simulink model "StudentClient_R2019b"  (R2019b)
settings: Solver=ode45  SolverName=VariableStepAuto  StartTime=0.0  StopTime=inf  FixedStep=1  RelTol=1e-3
undefined symbols (not defined in the file): f, gray
libraries: instrumentlib x3
settings Model: Creator=花舞  LastModifiedBy=admin
settings OptimizationCC: OptimizeBlockIOStorage=off  OptimizeDataStoreBuffers=off  BusAssignmentInplaceUpdate=off
settings DebuggingCC: SFUnexpectedBacktrackingDiag=warning  SFNoUnconditionalDefaultTransitionDiag=warning
settings RTWCC: GenerateReport=on  BuildConfiguration=Debug  LaunchReport=on
settings CodeAppCC: ForceParamTrailComments=on  MATLABSourceComments=on  EnableCustomComments=on
settings GRTTargetCC: CombineSignalStateStructs=on  SupportVariableSizeSignals=on  MultiInstanceErrorCode=Warning

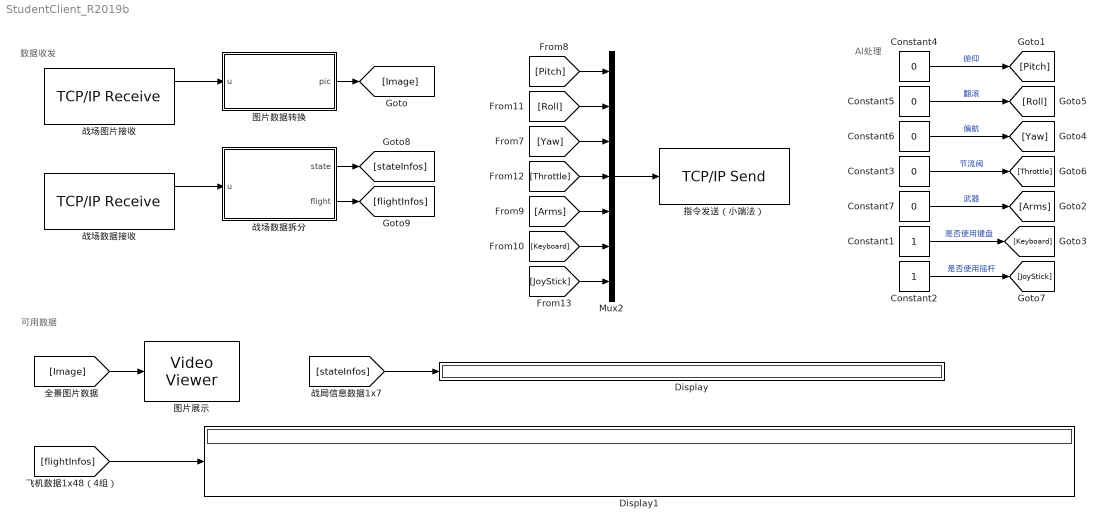
== system StudentClient_R2019b ==
  note: AI处理
  note: 可用数据
  note: 数据收发
  Constant1 : Constant  OutDataTypeStr=int32
  Constant2 : Constant  OutDataTypeStr=int32
  Constant{3..7} (5 alike) : Constant  Value=0  OutDataTypeStr=int32
  Display : Display
  Display1 : Display
  Mux2 : Mux  Inputs=7
  图片展示 : VideoViewer  colormapValue=gray(256)  FigPos=[1 1038 1920 937]
  图片数据转换 : MATLAB Function  TreatAsAtomicUnit=on
  战场图片接收 : instrumentlib/TCP//IP Receive  Host=0.0.0.0  Port=9999  DataSize="[1  1572864]"  EnableBlockingMode=off  Timeout=10  SampleTime=0.01  DataType=uint8  ByteOrder=BigEndian  ASCIIFormatting=%f,  Terminator=LF
  战场数据拆分 : MATLAB Function  TreatAsAtomicUnit=on
  战场数据接收 : instrumentlib/TCP//IP Receive  Host=0.0.0.0  Port=10000  DataSize="[1  55]"  EnableBlockingMode=off  Timeout=10  SampleTime=0.01  DataType=int32  ByteOrder=LittleEndian  ASCIIFormatting=%f,  Terminator=LF
  指令发送（小端法） : instrumentlib/TCP//IP Send  Host=0.0.0.0  Port=9999  EnableBlockingMode=off  Timeout=10  ByteOrder=LittleEndian  TransferDelay=on
  wires:
  战场图片接收/1 -> 图片数据转换/1(u)
  Constant4/1 -> [Pitch]  "俯仰"
  Constant5/1 -> [Roll]  "翻滚"
  Constant6/1 -> [Yaw]  "偏航"
  Constant3/1 -> [Throttle]  "节流阀"
  Constant7/1 -> [Arms]  "武器"
  Constant1/1 -> [Keyboard]  "是否使用键盘"
  Constant2/1 -> [JoyStick]  "是否使用摇杆"
  [Keyboard] -> Mux2/6
  [Roll] -> Mux2/2
  [Pitch] -> Mux2/1
  [Throttle] -> Mux2/4
  [Yaw] -> Mux2/3
  [Arms] -> Mux2/5
  [JoyStick] -> Mux2/7
  Mux2/1 -> 指令发送（小端法）/1
  图片数据转换/1(pic) -> [Image]
  [Image] -> 图片展示/1
  [stateInfos] -> Display/1
  [flightInfos] -> Display1/1
  战场数据接收/1 -> 战场数据拆分/1(u)
  战场数据拆分/1(state) -> [stateInfos]
  战场数据拆分/2(flight) -> [flightInfos]

== matlab function StudentClient_R2019b/图片数据转换 ==
  data: u input; pic output
function pic = fcn(u)
coder.extrinsic('image');
col = 1024;
row = 512;
temp = 1;
I = zeros(row, col, 3);
for i=1:row
    for j=1:col
        I(513 - i,j,1)=u(temp);
        I(513 - i,j,2)=u(temp+1);
        I(513 - i,j,3)=u(temp+2);
        temp = temp + 3;
    end
end
pic = double(I)/255;

== matlab function StudentClient_R2019b/战场数据拆分 ==
  data: u input; state output; flight output
function [state,flight] = fcn(u)
state = u(1:7);
flight = u(8:end);
